simulink model "k1visbsmon"  (Simulink 8.6)
settings: Solver=VariableStepAuto  StartTime=0.0  StopTime=10.0  RelTol=1e-3
libraries: cdsTP x10, cdsEpicsOut x10, cdsFilt x2, cdsAdcx0 x1, cdsParameters x1
settings Model: Creator=controls  LastModifiedBy=controls
settings DataIOCC: SaveFormat=Dataset  SignalLoggingSaveFormat=Dataset
settings OptimizationCC: ExpressionDepthLimit=128
settings DebuggingCC: UnderspecifiedInitializationDetection=Simplified  MergeDetectMultiDrivingBlocksExec=error  SolverPrmCheckMsg=none  FcnCallInpInsideContextMsg=EnableAllAsError  StateNameClashWarn=none
settings HardwareCC: ProdBitPerPointer=64  ProdLargestAtomicFloat=Float  ProdIntDivRoundTo=Zero  ProdEndianess=LittleEndian  ProdWordSize=64  ProdHWDeviceType=Intel->x86-64 (Windows64)
settings GRTTargetCC: GeneratePreprocessorConditionals=Use local settings  CombineOutputUpdateFcns=on  GRTInterface=off
settings ConfigComp: CovModelRefEnable=off

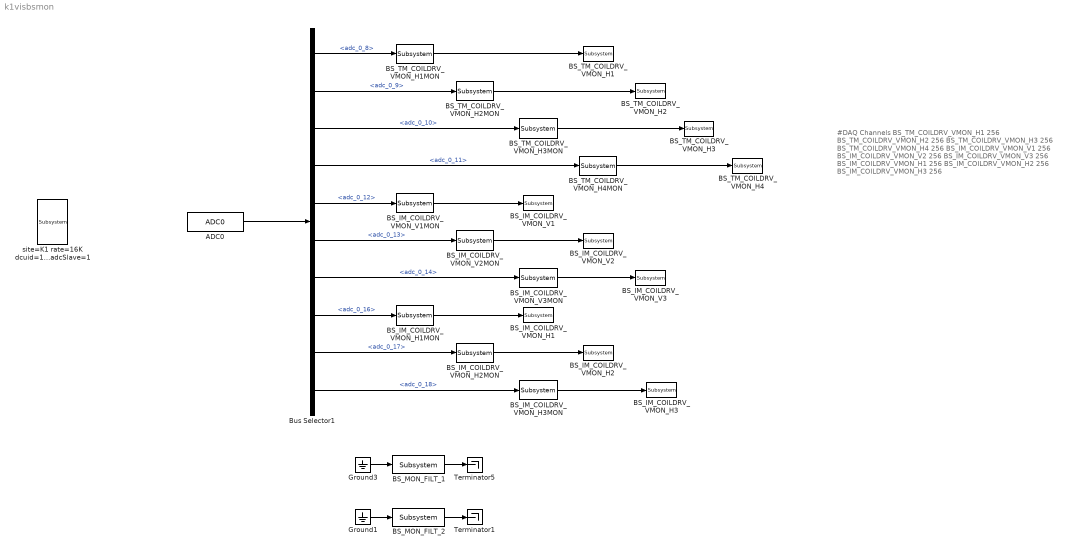
== system k1visbsmon ==
  note: #DAQ Channels
      |
      | BS_TM_COILDRV_VMON_H1 256
      | BS_TM_COILDRV_VMON_H2 256
      | BS_TM_COILDRV_VMON_H3 256
      | BS_TM_COILDRV_VMON_H4 256
      | BS_IM_COILDRV_VMON_V1 256
      | BS_IM_COILDRV_VMON_V2 256
      | BS_IM_COILDRV_VMON_V3 256
      | BS_IM_COILDRV_VMON_H1 256
      | BS_IM_COILDRV_VMON_H2 256
      | BS_IM_COILDRV_VMON_H3 256
  ADC0 : cdsAdcx0/ADC0  Tag=cdsAdc  Description=|
      | type-GSC_16AI64SSA
      | card_num=0
      settings: AttributesFormatString=%<Description>\n%<Tag>
  BS_IM_COILDRV_VMON_H1 : cdsTP/Subsystem  Tag=Test Point
      settings: AttributesFormatString=%<Tag>
  BS_IM_COILDRV_VMON_H1MON : cdsEpicsOut/Subsystem  Tag=cdsEpicsOutput  Description=|
      | Purpose:                                          
      | Output a FE signal to an EPICS channel.           
      |                                                   
      | Operation:                                        
      | Takes input value and passes it to EPICS record.  
      |                                                   
      | Usage:                                            
      | Name the part with the desired EPICS rrecord name.
      settings: AttributesFormatString=%<Tag>
  BS_IM_COILDRV_VMON_H2 : cdsTP/Subsystem  Tag=Test Point
      settings: AttributesFormatString=%<Tag>
  BS_IM_COILDRV_VMON_H2MON : cdsEpicsOut/Subsystem  Tag=cdsEpicsOutput  Description=|
      | Purpose:                                          
      | Output a FE signal to an EPICS channel.           
      |                                                   
      | Operation:                                        
      | Takes input value and passes it to EPICS record.  
      |                                                   
      | Usage:                                            
      | Name the part with the desired EPICS rrecord name.
      settings: AttributesFormatString=%<Tag>
  BS_IM_COILDRV_VMON_H3 : cdsTP/Subsystem  Tag=Test Point
      settings: AttributesFormatString=%<Tag>
  BS_IM_COILDRV_VMON_H3MON : cdsEpicsOut/Subsystem  Tag=cdsEpicsOutput  Description=|
      | Purpose:                                          
      | Output a FE signal to an EPICS channel.           
      |                                                   
      | Operation:                                        
      | Takes input value and passes it to EPICS record.  
      |                                                   
      | Usage:                                            
      | Name the part with the desired EPICS rrecord name.
      settings: AttributesFormatString=%<Tag>
  BS_IM_COILDRV_VMON_V1 : cdsTP/Subsystem  Tag=Test Point
      settings: AttributesFormatString=%<Tag>
  BS_IM_COILDRV_VMON_V1MON : cdsEpicsOut/Subsystem  Tag=cdsEpicsOutput  Description=|
      | Purpose:                                          
      | Output a FE signal to an EPICS channel.           
      |                                                   
      | Operation:                                        
      | Takes input value and passes it to EPICS record.  
      |                                                   
      | Usage:                                            
      | Name the part with the desired EPICS rrecord name.
      settings: AttributesFormatString=%<Tag>
  BS_IM_COILDRV_VMON_V2 : cdsTP/Subsystem  Tag=Test Point
      settings: AttributesFormatString=%<Tag>
  BS_IM_COILDRV_VMON_V2MON : cdsEpicsOut/Subsystem  Tag=cdsEpicsOutput  Description=|
      | Purpose:                                          
      | Output a FE signal to an EPICS channel.           
      |                                                   
      | Operation:                                        
      | Takes input value and passes it to EPICS record.  
      |                                                   
      | Usage:                                            
      | Name the part with the desired EPICS rrecord name.
      settings: AttributesFormatString=%<Tag>
  BS_IM_COILDRV_VMON_V3 : cdsTP/Subsystem  Tag=Test Point
      settings: AttributesFormatString=%<Tag>
  BS_IM_COILDRV_VMON_V3MON : cdsEpicsOut/Subsystem  Tag=cdsEpicsOutput  Description=|
      | Purpose:                                          
      | Output a FE signal to an EPICS channel.           
      |                                                   
      | Operation:                                        
      | Takes input value and passes it to EPICS record.  
      |                                                   
      | Usage:                                            
      | Name the part with the desired EPICS rrecord name.
      settings: AttributesFormatString=%<Tag>
  BS_MON_FILT_1 : cdsFilt/Subsystem  Tag=cdsFilt  Description=|
      | Purpose:                                                                                                                                                                                                                                  
      | Standard CDS IIR filter module.                                                                                                                                                                                                           
      |                                                                                                                                                                                                                                           
      | Operation:                                                                                                                                                                                                                                
      | Consists of 10 second order section IIR filters, plus a ramped gain stage. In FE code, also provides pre-defined test points and excitation channel inputs. The filter coefficients are defined in the LIGO system using the 'foton' tool.
      |                                                                                                                                                                                                                                           
      | Usage:                                                                                                                                                                                                                                    
      | Name the part with the desired filter module name.
      settings: AttributesFormatString=%<Tag>
  BS_MON_FILT_2 : cdsFilt/Subsystem  Tag=cdsFilt  Description=|
      | Purpose:                                                                                                                                                                                                                                  
      | Standard CDS IIR filter module.                                                                                                                                                                                                           
      |                                                                                                                                                                                                                                           
      | Operation:                                                                                                                                                                                                                                
      | Consists of 10 second order section IIR filters, plus a ramped gain stage. In FE code, also provides pre-defined test points and excitation channel inputs. The filter coefficients are defined in the LIGO system using the 'foton' tool.
      |                                                                                                                                                                                                                                           
      | Usage:                                                                                                                                                                                                                                    
      | Name the part with the desired filter module name.
      settings: AttributesFormatString=%<Tag>
  BS_TM_COILDRV_VMON_H{1..4} (4 alike) : cdsTP/Subsystem  Tag=Test Point
      settings: AttributesFormatString=%<Tag>
  BS_TM_COILDRV_VMON_H1MON : cdsEpicsOut/Subsystem  Tag=cdsEpicsOutput  Description=|
      | Purpose:                                          
      | Output a FE signal to an EPICS channel.           
      |                                                   
      | Operation:                                        
      | Takes input value and passes it to EPICS record.  
      |                                                   
      | Usage:                                            
      | Name the part with the desired EPICS rrecord name.
      settings: AttributesFormatString=%<Tag>
  BS_TM_COILDRV_VMON_H2MON : cdsEpicsOut/Subsystem  Tag=cdsEpicsOutput  Description=|
      | Purpose:                                          
      | Output a FE signal to an EPICS channel.           
      |                                                   
      | Operation:                                        
      | Takes input value and passes it to EPICS record.  
      |                                                   
      | Usage:                                            
      | Name the part with the desired EPICS rrecord name.
      settings: AttributesFormatString=%<Tag>
  BS_TM_COILDRV_VMON_H3MON : cdsEpicsOut/Subsystem  Tag=cdsEpicsOutput  Description=|
      | Purpose:                                          
      | Output a FE signal to an EPICS channel.           
      |                                                   
      | Operation:                                        
      | Takes input value and passes it to EPICS record.  
      |                                                   
      | Usage:                                            
      | Name the part with the desired EPICS rrecord name.
      settings: AttributesFormatString=%<Tag>
  BS_TM_COILDRV_VMON_H4MON : cdsEpicsOut/Subsystem  Tag=cdsEpicsOutput  Description=|
      | Purpose:                                          
      | Output a FE signal to an EPICS channel.           
      |                                                   
      | Operation:                                        
      | Takes input value and passes it to EPICS record.  
      |                                                   
      | Usage:                                            
      | Name the part with the desired EPICS rrecord name.
      settings: AttributesFormatString=%<Tag>
  Bus Selector1 : BusSelector  Description=ADC Selector  OutputSignals=adc_0_8,adc_0_9,adc_0_10,adc_0_11,adc_0_12,adc_0_13,adc_0_14,adc_0_16,adc_0_17,adc_0_18
      settings: AttributesFormatString=%<Description>
  Ground1 : Ground
  Ground3 : Ground
  Terminator1 : Terminator
  Terminator5 : Terminator
  site=K1 rate=16K dcuid=1094 host=k1asc0 specific_cpu=4 adcSlave=1 : cdsParameters/Subsystem  Tag=cdsParameters  Description=|
      | Purpose:                                                                                                                                                                                                                                
      | Provide system parameters to the FE code generator to properly configure the generated EPICS names, rep rate of the FE controller, and the Data Acquisition node ID for proper storage of data from this FE controller.                 
      |                                                                                                                                                                                                                                         
      | Useage:                                                                                                                                                                                                                                 
      | The part NAME field is used to identify the FE parameters. It must be of the form:                                                                                                                                                      
      | site=                                                                                                                                                                                                                                   
      | rate=                                                                                                                                                                                                                                   
      | dcuid=                                                                                                                                                                                                                                  
      |                                                                                                                                                                                                                                         
      | Where:                                                                                                                                                                                                                                  
      | site= argument may be H1, H2, L1, M1, G1, either as a single argument or multiple, for example site=H1,H2. These are the only names allowed. These will become the first two characters of all EPICS and signal names (for example G1:).
      |                                                                                                                                                                                                                                         
      | rate= may be 2K, 16K, 32K, or 64K                                                                                                                                                                                                       
      |                                                                                                                                                                                                                                         
      | dcuid= is site specific ie it must be unique at each site.
      settings: AttributesFormatString=%<Tag>
  wires:
  ADC0/1 -> Bus Selector1/1
  Bus Selector1/1 -> BS_TM_COILDRV_VMON_H1MON/1  "<adc_0_8>"
  BS_TM_COILDRV_VMON_H1MON/1 -> BS_TM_COILDRV_VMON_H1/1
  BS_TM_COILDRV_VMON_H2MON/1 -> BS_TM_COILDRV_VMON_H2/1
  Bus Selector1/2 -> BS_TM_COILDRV_VMON_H2MON/1  "<adc_0_9>"
  BS_TM_COILDRV_VMON_H3MON/1 -> BS_TM_COILDRV_VMON_H3/1
  BS_TM_COILDRV_VMON_H4MON/1 -> BS_TM_COILDRV_VMON_H4/1
  Bus Selector1/4 -> BS_TM_COILDRV_VMON_H4MON/1  "<adc_0_11>"
  Bus Selector1/3 -> BS_TM_COILDRV_VMON_H3MON/1  "<adc_0_10>"
  BS_IM_COILDRV_VMON_V1MON/1 -> BS_IM_COILDRV_VMON_V1/1
  Bus Selector1/5 -> BS_IM_COILDRV_VMON_V1MON/1  "<adc_0_12>"
  BS_IM_COILDRV_VMON_V2MON/1 -> BS_IM_COILDRV_VMON_V2/1
  Bus Selector1/6 -> BS_IM_COILDRV_VMON_V2MON/1  "<adc_0_13>"
  BS_IM_COILDRV_VMON_V3MON/1 -> BS_IM_COILDRV_VMON_V3/1
  Bus Selector1/7 -> BS_IM_COILDRV_VMON_V3MON/1  "<adc_0_14>"
  BS_IM_COILDRV_VMON_H1MON/1 -> BS_IM_COILDRV_VMON_H1/1
  Bus Selector1/8 -> BS_IM_COILDRV_VMON_H1MON/1  "<adc_0_16>"
  BS_IM_COILDRV_VMON_H2MON/1 -> BS_IM_COILDRV_VMON_H2/1
  Bus Selector1/9 -> BS_IM_COILDRV_VMON_H2MON/1  "<adc_0_17>"
  BS_IM_COILDRV_VMON_H3MON/1 -> BS_IM_COILDRV_VMON_H3/1
  Bus Selector1/10 -> BS_IM_COILDRV_VMON_H3MON/1  "<adc_0_18>"
  Ground3/1 -> BS_MON_FILT_1/1
  Ground1/1 -> BS_MON_FILT_2/1
  BS_MON_FILT_1/1 -> Terminator5/1
  BS_MON_FILT_2/1 -> Terminator1/1
